simulink model "CCH_EMF_LIN"  (R2023a)
settings: Solver=VariableStepAuto  StartTime=0.0  StopTime=10.0  RelTol=1e-3
values from neighbouring files (symbols this model uses):
  AA = tlr{1}    [initLinCCH6dof.m]    (also in initalizeLinearCCH.m)
  BB = tlr{2}    [initLinCCH6dof.m]    (also in initalizeLinearCCH.m)
  CC = tlr{3}    [initLinCCH6dof.m]    (also in initalizeLinearCCH.m)
  DD = tlr{4}    [initLinCCH6dof.m]    (also in initalizeLinearCCH.m)
  epsilon = 0.0000001    (= 1e-07)    [coaxial_heli_parameters.m]    (also in nonLinearSimulation.m = 0.001)
  M_delta_e = TrimLinSave{idx_speed,2}(3,4)    [EMFController3dofSimulation3211.m]    (also in EMFController6dofSimulationBobAccelDecell.m = TrimLinSave_6dof{idx_speed,2}(5,7); initLinCCH6dof.m = BB(5,7); initalizeLinearCCH.m = BB(3,4); nonLimSimFunction.m = TrimLinSave_6dof{idx_speed,2}(5,7))
  M_theta_s = TrimLinSave_6dof{idx_speed,2}(5,3)    [EMFController6dofSimulationBobAccelDecell.m]    (also in initLinCCH6dof.m = BB(5,3); initalizeLinearCCH.m = BB(3,2); nonLimSimFunction.m)
  V_l_transit = V_transit_save(1)    [EMFController3dofSimulation3211.m]    (also in EMFController6dofSimulationBobAccelDecell.m = V_transit_save(1)/1.94384; initLinCCH6dof.m; initalizeLinearCCH.m; nonLimSimFunction.m)
  V_u_transit = V_transit_save(2)-20    [EMFController3dofSimulation3211.m]    (also in EMFController6dofSimulationBobAccelDecell.m = V_transit_save(2)/1.94384-20; initLinCCH6dof.m = V_transit_save(2); initalizeLinearCCH.m = V_transit_save(2); nonLimSimFunction.m)
libraries: simulink_extras x4, slpidlib x2, SignalEditorBlockLib x1
settings Model: Creator=prenc  LastModifiedBy=prenc

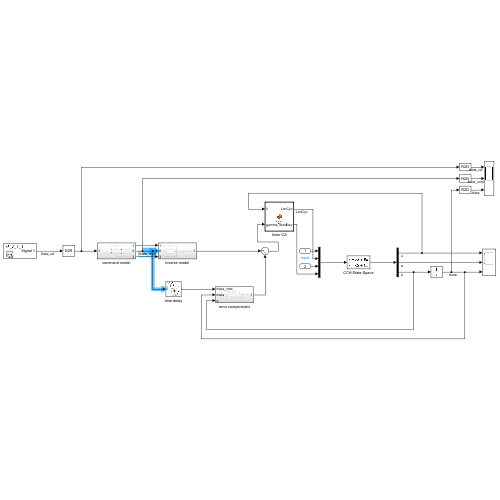
[thumbnail: Simulink's stored preview of the top-level diagram]
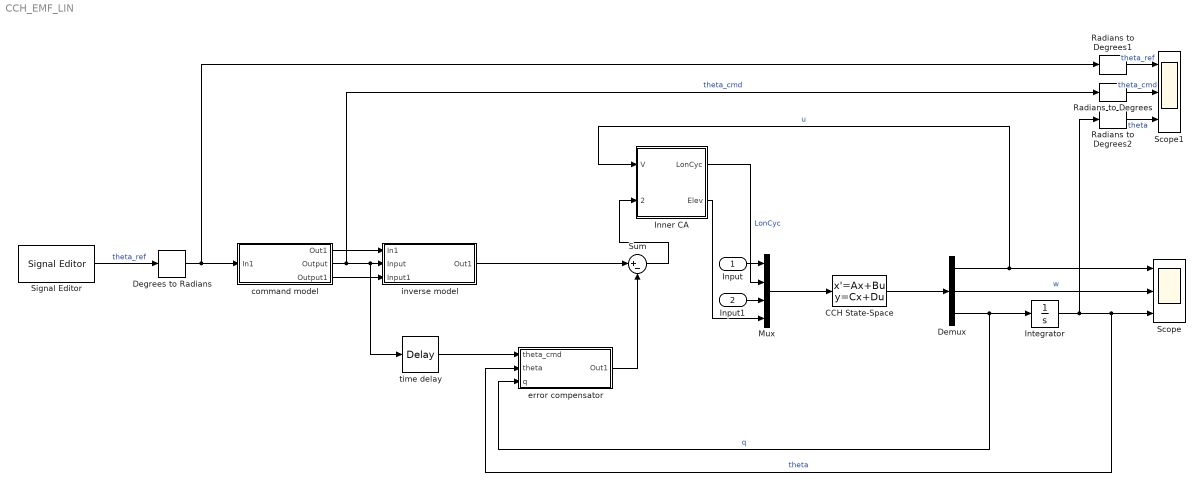
== system CCH_EMF_LIN ==
  Input : Inport
  Input1 : Inport  Port=2
  CCH State-Space : StateSpace  A=AA  B=BB  C=CC  D=DD  InitialCondition=0
  Degrees to Radians : simulink_extras/Transformations/Degrees to Radians
  Demux : Demux  Outputs=3
  Inner CA : MATLAB Function  TreatAsAtomicUnit=on
  Integrator : Integrator
  Mux : Mux
  Radians to Degrees : simulink_extras/Transformations/Radians to Degrees
  Radians to Degrees1 : simulink_extras/Transformations/Radians to Degrees
  Radians to Degrees2 : simulink_extras/Transformations/Radians to Degrees
  Scope : Scope  NumInputPorts=3
  Scope1 : Scope  NumInputPorts=3
  Signal Editor : SignalEditorBlockLib/Signal Editor  FileName=C:\Users\prenc\Documents\GitHub\CCHThesis\Generated Signals Simulink\3-2-1-1.mat  ActiveScenario=x3_2_1_1  ActiveSignal=Signal 1  IsBus=off  OutputBusObjectStr=Bus: BusObject  SampleTime=0  Interpolate=off  ZeroCross=off  OutputAfterFinalValue=Setting to zero  Unit=inherit  PreserveSignalName=on  ApplySigPropsToAllScenarios=on
  Sum : Sum  Inputs=|+-
  command model : Subsystem
  error compensator : Subsystem
  inverse model : Subsystem
  time delay : TransportDelay  DelayTime=0.12
  wires:
  CCH State-Space/1 -> Demux/1
  Mux/1 -> CCH State-Space/1
  Signal Editor/1 -> Degrees to Radians/1  "theta_ref"
  command model/1(Out1) -> inverse model/1(In1)
  command model/2(Output) -> Radians to Degrees/1, time delay/1, inverse model/2(Input)  "theta_cmd"
  command model/3(Output1) -> inverse model/3(Input1)
  inverse model/1(Out1) -> Sum/1
  time delay/1 -> error compensator/1(theta_cmd)
  error compensator/1(Out1) -> Sum/2
  Demux/1 -> Inner CA/1(V), Scope/1  "u"
  Demux/2 -> Scope/2  "w"
  Demux/3 -> Integrator/1, error compensator/3(q)  "q"
  Integrator/1 -> Radians to Degrees2/1, Scope/3, error compensator/2(theta)  "theta"
  Input/1 -> Mux/1
  Input1/1 -> Mux/3
  Inner CA/2(Elev) -> Mux/4
  Degrees to Radians/1 -> Radians to Degrees1/1, command model/1(In1)
  Radians to Degrees/1 -> Scope1/2  "theta_cmd"
  Radians to Degrees1/1 -> Scope1/1  "theta_ref"
  Radians to Degrees2/1 -> Scope1/3  "theta"
  Inner CA/1(LonCyc) -> Mux/2  "LonCyc"
  Sum/1 -> Inner CA/2(gamma_theta)

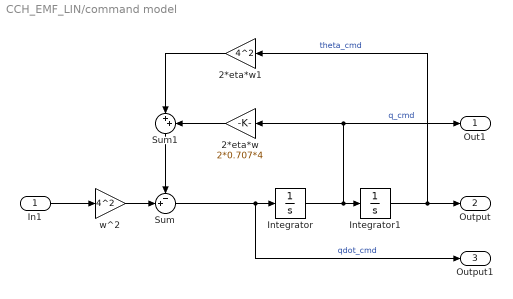
== system CCH_EMF_LIN/command model ==
  In1 : Inport
  2*eta*w : Gain  Gain=2*0.707*4
  2*eta*w1 : Gain  Gain=4^2
  Integrator : Integrator
  Integrator1 : Integrator
  Sum : Sum  Inputs=-+|
  Sum1 : Sum  Inputs=|++
  w^2 : Gain  Gain=4^2
  Out1 : Outport
  Output : Outport  Port=2
  Output1 : Outport  Port=3
  wires:
  In1/1 -> w^2/1
  w^2/1 -> Sum/2
  Sum1/1 -> Sum/1
  2*eta*w/1 -> Sum1/2
  2*eta*w1/1 -> Sum1/1
  Sum/1 -> Output1/1, Integrator/1  "qdot_cmd"
  Integrator/1 -> 2*eta*w/1, Out1/1, Integrator1/1  "q_cmd"
  Integrator1/1 -> 2*eta*w1/1, Output/1  "theta_cmd"

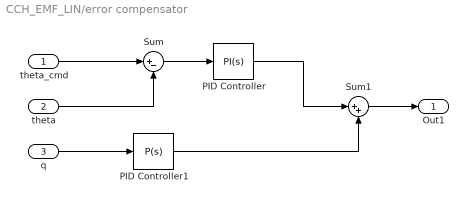
== system CCH_EMF_LIN/error compensator ==
  theta_cmd : Inport
  theta : Inport  Port=2
  q : Inport  Port=3
  PID Controller : slpidlib/PID Controller  Controller=PI  Form=Parallel  TimeDomain=Continuous-time  UseExternalTs=off  SampleTime=-1  IntegratorMethod=Forward Euler  FilterMethod=Forward Euler  ControllerParametersSource=internal  P=-13.2157554586336  I=-2.52197272765188  UseKiTs=off  D=0  N=100  UseFilter=on  TunerSelectOption=Transfer Function Based (PID Tuner App)  InitialConditionSource=internal  InitialConditionForIntegrator=0  InitialConditionForFilter=0  DifferentiatorICPrevScaledInput=0  ExternalReset=none  TrackingMode=off  Kt=1  LimitOutput=off  SatLimitsSource=internal  UpperSaturationLimit=inf  LowerSaturationLimit=-inf  LinearizeAsGain=on  AntiWindupMode=none  Kb=1  LimitIntegrator=off  UpperIntegratorSaturationLimit=inf  LowerIntegratorSaturationLimit=-inf  POutMin=[]  POutMax=[]  IOutMin=[]  IOutMax=[]  DOutMin=[]  DOutMax=[]  NOutMin=[]  NOutMax=[]  SumOutMin=[]  SumOutMax=[]  SaturationOutMin=[]  SaturationOutMax=[]  PParamMin=[]  PParamMax=[]  IParamMin=[]  IParamMax=[]  DParamMin=[]  DParamMax=[]  NParamMin=[]  NParamMax=[]  KbParamMin=[]  KbParamMax=[]  KtParamMin=[]  KtParamMax=[]  KbOutMin=[]  KbOutMax=[]  KtOutMin=[]  KtOutMax=[]  IntegratorOutMin=[]  IntegratorOutMax=[]  FilterOutMin=[]  FilterOutMax=[]  SumI1OutMin=[]  SumI1OutMax=[]  SumI2OutMin=[]  SumI2OutMax=[]  SumI3OutMin=[]  SumI3OutMax=[]  SumI4OutMin=[]  SumI4OutMax=[]  SumDOutMin=[]  SumDOutMax=[]  DifferentiatorOutMin=[]  DifferentiatorOutMax=[]  FilterDiffOutCoefMin=[]  FilterDiffOutCoefMax=[]  ReciprocalOutMin=[]  ReciprocalOutMax=[]  SumDenOutMin=[]  SumDenOutMax=[]  SumNumOutMin=[]  SumNumOutMax=[]  DivideOutMin=[]  DivideOutMax=[]  UdiffTsProdOutMin=[]  UdiffTsProdOutMax=[]  NTsProdOutMin=[]  NTsProdOutMax=[]  UintegralTsProdOutMin=[]  UintegralTsProdOutMax=[]  UngainTsProdOutMin=[]  UngainTsProdOutMax=[]  ClampingZeroOutDataTypeStr=Inherit: Inherit via back propagation  ClampingZeroOutMin=[]  ClampingZeroOutMax=[]  FilterDenConstantOutDataTypeStr=Inherit: Inherit via back propagation  FilterDenConstantOutMin=[]  FilterDenConstantOutMax=[]  PCopyOutDataTypeStr=Inherit: Inherit via back propagation  PCopyOutMin=[]  PCopyOutMax=[]  NCopyOutDataTypeStr=Inherit: Inherit via back propagation  NCopyOutMin=[]  NCopyOutMax=[]  IntegratorContinuousStateAttributes=''  IntegratorStateMustResolveToSignalObject=off  IntegratorRTWStateStorageClass=Auto  FilterContinuousStateAttributes=''  FilterStateMustResolveToSignalObject=off  FilterRTWStateStorageClass=Auto  ParallelPVariant=InternalParameters  IdealPVariant=Disabled  IVariant=InternalParameters  DVariant=Disabled  IntegratorVariant=Continuous  SatVariant=Disabled  AWVariant=Passthrough  PCopyVariant=Disabled  TRVariant=Disabled  FdbkBlocksVariant=Forward  IdealPFdbkVariant=Disabled  SatFdbkVariant=Disabled  DerivativeFilterVariant=Disabled  NVariant=Disabled  NCopyVariant=Disabled_SignalSpec  FilterICVariant=Disabled  IntegratorICVariant=InternalICs  ExternalResetVariant=Disabled  TRSumVariant=Passthrough  SumFdbkVariant=Disabled  SumVariant=Sum_PI  TsampFilterVariant=InternalTs  TsampNgainVariant=Passthrough  TsampIntegralVariant=Disabled_SignalSpec  ExternalSaturationOutDataTypeStr=Inherit: Same as second input
  PID Controller1 : slpidlib/PID Controller  Controller=P  Form=Parallel  TimeDomain=Continuous-time  UseExternalTs=off  SampleTime=-1  IntegratorMethod=Forward Euler  FilterMethod=Forward Euler  ControllerParametersSource=internal  P=31.9331440525019  I=1.2  UseKiTs=off  D=0  N=100  UseFilter=on  TunerSelectOption=Transfer Function Based (PID Tuner App)  InitialConditionSource=internal  InitialConditionForIntegrator=0  InitialConditionForFilter=0  DifferentiatorICPrevScaledInput=0  ExternalReset=none  TrackingMode=off  Kt=1  LimitOutput=off  SatLimitsSource=internal  UpperSaturationLimit=inf  LowerSaturationLimit=-inf  LinearizeAsGain=on  AntiWindupMode=none  Kb=1  LimitIntegrator=off  UpperIntegratorSaturationLimit=inf  LowerIntegratorSaturationLimit=-inf  POutMin=[]  POutMax=[]  IOutMin=[]  IOutMax=[]  DOutMin=[]  DOutMax=[]  NOutMin=[]  NOutMax=[]  SumOutMin=[]  SumOutMax=[]  SaturationOutMin=[]  SaturationOutMax=[]  PParamMin=[]  PParamMax=[]  IParamMin=[]  IParamMax=[]  DParamMin=[]  DParamMax=[]  NParamMin=[]  NParamMax=[]  KbParamMin=[]  KbParamMax=[]  KtParamMin=[]  KtParamMax=[]  KbOutMin=[]  KbOutMax=[]  KtOutMin=[]  KtOutMax=[]  IntegratorOutMin=[]  IntegratorOutMax=[]  FilterOutMin=[]  FilterOutMax=[]  SumI1OutMin=[]  SumI1OutMax=[]  SumI2OutMin=[]  SumI2OutMax=[]  SumI3OutMin=[]  SumI3OutMax=[]  SumI4OutMin=[]  SumI4OutMax=[]  SumDOutMin=[]  SumDOutMax=[]  DifferentiatorOutMin=[]  DifferentiatorOutMax=[]  FilterDiffOutCoefMin=[]  FilterDiffOutCoefMax=[]  ReciprocalOutMin=[]  ReciprocalOutMax=[]  SumDenOutMin=[]  SumDenOutMax=[]  SumNumOutMin=[]  SumNumOutMax=[]  DivideOutMin=[]  DivideOutMax=[]  UdiffTsProdOutMin=[]  UdiffTsProdOutMax=[]  NTsProdOutMin=[]  NTsProdOutMax=[]  UintegralTsProdOutMin=[]  UintegralTsProdOutMax=[]  UngainTsProdOutMin=[]  UngainTsProdOutMax=[]  ClampingZeroOutDataTypeStr=Inherit: Inherit via back propagation  ClampingZeroOutMin=[]  ClampingZeroOutMax=[]  FilterDenConstantOutDataTypeStr=Inherit: Inherit via back propagation  FilterDenConstantOutMin=[]  FilterDenConstantOutMax=[]  PCopyOutDataTypeStr=Inherit: Inherit via back propagation  PCopyOutMin=[]  PCopyOutMax=[]  NCopyOutDataTypeStr=Inherit: Inherit via back propagation  NCopyOutMin=[]  NCopyOutMax=[]  IntegratorContinuousStateAttributes=''  IntegratorStateMustResolveToSignalObject=off  IntegratorRTWStateStorageClass=Auto  FilterContinuousStateAttributes=''  FilterStateMustResolveToSignalObject=off  FilterRTWStateStorageClass=Auto  ParallelPVariant=InternalParameters  IdealPVariant=Disabled  IVariant=Disabled  DVariant=Disabled  IntegratorVariant=Disabled  SatVariant=Disabled  AWVariant=Disabled  PCopyVariant=Disabled  TRVariant=Disabled  FdbkBlocksVariant=Forward  IdealPFdbkVariant=Disabled  SatFdbkVariant=Disabled  DerivativeFilterVariant=Disabled  NVariant=Disabled  NCopyVariant=Disabled_SignalSpec  FilterICVariant=Disabled  IntegratorICVariant=Disabled  ExternalResetVariant=Disabled  TRSumVariant=Passthrough  SumFdbkVariant=Disabled  SumVariant=Passthrough_P  TsampFilterVariant=InternalTs  TsampNgainVariant=Passthrough  TsampIntegralVariant=Disabled_SignalSpec  ExternalSaturationOutDataTypeStr=Inherit: Same as second input
  Sum : Sum  Inputs=|+-
  Sum1 : Sum  Inputs=|++
  Out1 : Outport
  wires:
  theta_cmd/1 -> Sum/1
  theta/1 -> Sum/2
  Sum/1 -> PID Controller/1
  q/1 -> PID Controller1/1
  PID Controller/1 -> Sum1/1
  PID Controller1/1 -> Sum1/2
  Sum1/1 -> Out1/1

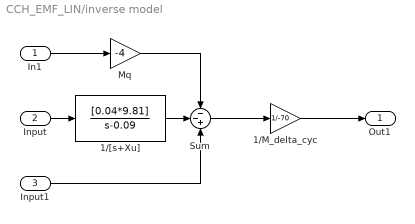
== system CCH_EMF_LIN/inverse model ==
  In1 : Inport
  Input : Inport  Port=2
  Input1 : Inport  Port=3
  1/M_delta_cyc : Gain  Gain=1/-70
  1/[s+Xu] : TransferFcn  Numerator=[0.04*9.81]  Denominator=[1 -0.09]
  Mq : Gain  Gain=-4
  Sum : Sum  Inputs=--+
  Out1 : Outport
  wires:
  In1/1 -> Mq/1
  Mq/1 -> Sum/1
  Input1/1 -> Sum/3
  1/M_delta_cyc/1 -> Out1/1
  Sum/1 -> 1/M_delta_cyc/1
  1/[s+Xu]/1 -> Sum/2
  Input/1 -> 1/[s+Xu]/1

== matlab function CCH_EMF_LIN/Inner CA ==
  data: V input; LonCyc output; gamma_theta input; Elev output; V_l_transit parameter; epsilon parameter; V_u_transit parameter; M_theta_s parameter; M_delta_e parameter
function [LonCyc, Elev] = fcn(V, gamma_theta, V_l_transit, epsilon, V_u_transit, M_theta_s, M_delta_e)
    
    % Allocation Weights
    if V<V_l_transit
        rho_theta_c = 1;
        rho_delta_e = epsilon;

    elseif V>V_l_transit && V<V_u_transit
        rho_theta_c = 1 - 1/(V_u_transit-V_l_transit)*(V-V_l_transit);
        rho_delta_e = 1/(V_u_transit-V_l_transit)*(V-V_l_transit);

    else
        rho_theta_c = epsilon;
        rho_delta_e = 1;

    end

    % Allocation
    B_theta = [M_theta_s, M_delta_e];
    W_theta = [1/rho_theta_c, 0; 0, 1/rho_delta_e];
    U_theta = inv(W_theta)*transpose(B_theta)*inv(B_theta*inv(W_theta)*transpose(B_theta))*gamma_theta;

    LonCyc = U_theta(1);
    Elev = U_theta(2);
